simulink model "temperatureSubsytem"  (R2024b)
settings: Solver=VariableStepAuto  StartTime=0.0  StopTime=10.0  RelTol=1e-3

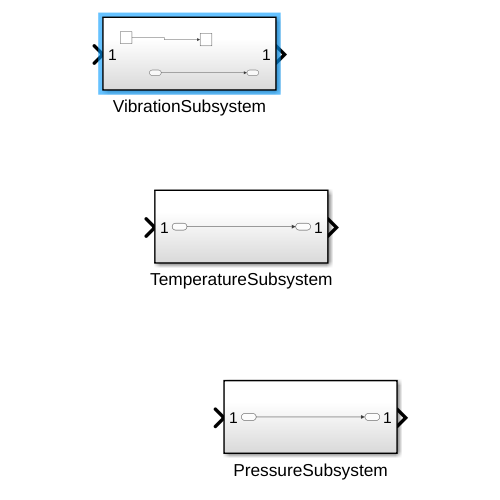
[thumbnail: Simulink's stored preview of the top-level diagram]
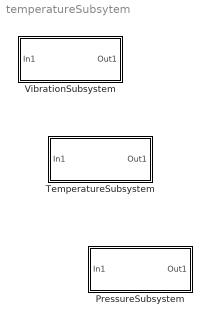
== system temperatureSubsytem ==
  PressureSubsystem : Subsystem
  TemperatureSubsystem : Subsystem
  VibrationSubsystem : Subsystem

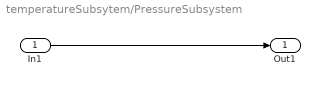
== system temperatureSubsytem/PressureSubsystem ==
  In1 : Inport
  Out1 : Outport
  wires:
  In1/1 -> Out1/1

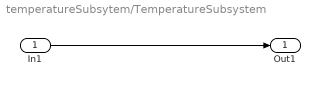
== system temperatureSubsytem/TemperatureSubsystem ==
  In1 : Inport
  Out1 : Outport
  wires:
  In1/1 -> Out1/1

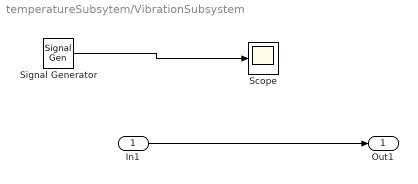
== system temperatureSubsytem/VibrationSubsystem ==
  In1 : Inport
  Scope : Scope
  Signal Generator : SignalGenerator  Units=rad/sec
  Out1 : Outport
  wires:
  In1/1 -> Out1/1
  Signal Generator/1 -> Scope/1
